simulink model "P_fuzzy"  (R2021a)
settings: Solver=VariableStepAuto  StartTime=0.0  StopTime=150  RelTol=1e-3
libraries: fuzblock x2
settings Model: Creator=Hang Dao  LastModifiedBy=Hang Dao

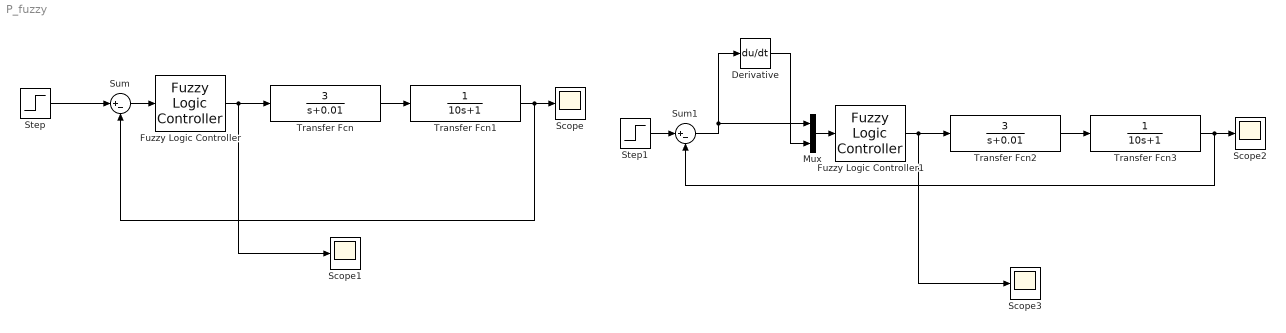
== system P_fuzzy ==
  Derivative : Derivative  CoefficientInTFapproximation=0.01
  Fuzzy Logic Controller : fuzblock/Fuzzy Logic  Controller  FIS='Pfuzzy.fis'  OutputSampleNumber=101  DataType=double  FuzzifiedInputs=off  RuleFiringStrengths=off  RuleOutputs=off  AggregatedOutputs=off  SimulateUsing=Interpreted execution  OutOfRangeInputValueMessage=warning  NoRuleFiredMessage=warning  EmptyOutputFuzzySetMessage=warning
  Fuzzy Logic Controller1 : fuzblock/Fuzzy Logic  Controller  FIS='Pfuzzy.fis'  OutputSampleNumber=101  DataType=double  FuzzifiedInputs=off  RuleFiringStrengths=off  RuleOutputs=off  AggregatedOutputs=off  SimulateUsing=Interpreted execution  OutOfRangeInputValueMessage=warning  NoRuleFiredMessage=warning  EmptyOutputFuzzySetMessage=warning
  Mux : Mux  Inputs=2
  Scope{,1..3} (4 alike) : Scope
  Step : Step  Time=0  SampleTime=0
  Step1 : Step  Time=0  SampleTime=0
  Sum : Sum  Inputs=|+-
  Sum1 : Sum  Inputs=|+-
  Transfer Fcn : TransferFcn  Numerator=[3]  Denominator=[1 0.01]
  Transfer Fcn1 : TransferFcn  Denominator=[10 1]
  Transfer Fcn2 : TransferFcn  Numerator=[3]  Denominator=[1 0.01]
  Transfer Fcn3 : TransferFcn  Denominator=[10 1]
  wires:
  Fuzzy Logic Controller/1 -> Scope1/1, Transfer Fcn/1
  Sum/1 -> Fuzzy Logic Controller/1
  Transfer Fcn/1 -> Transfer Fcn1/1
  Step/1 -> Sum/1
  Transfer Fcn1/1 -> Scope/1, Sum/2
  Transfer Fcn2/1 -> Transfer Fcn3/1
  Transfer Fcn3/1 -> Scope2/1, Sum1/2
  Fuzzy Logic Controller1/1 -> Scope3/1, Transfer Fcn2/1
  Step1/1 -> Sum1/1
  Mux/1 -> Fuzzy Logic Controller1/1
  Sum1/1 -> Mux/1, Derivative/1
  Derivative/1 -> Mux/2
